simulink model "PID_controlinput_tracking"  (R2022a)
settings: Solver=VariableStepAuto  StartTime=0.0  StopTime=10  RelTol=1e-3
libraries: cstblocks x2
settings Model: Creator=Linxi Ren  LastModifiedBy=Linxi Ren

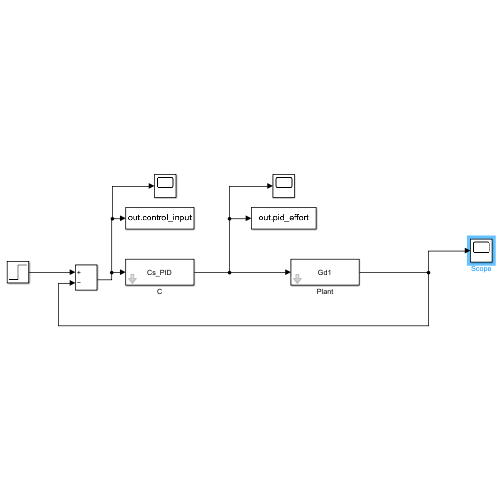
[thumbnail: Simulink's stored preview of the top-level diagram]
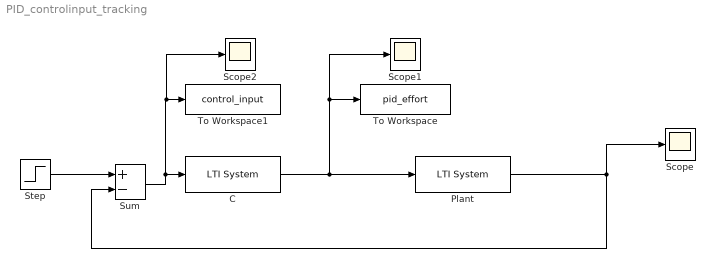
== system PID_controlinput_tracking ==
  C : cstblocks/LTI System  sys=Cs_PID  IC=[]
  Plant : cstblocks/LTI System  sys=Gd1  IC=[]
  Scope : Scope
  Scope1 : Scope
  Scope2 : Scope
  Step : Step  Time=0  SampleTime=0.0325
  Sum : Sum  Inputs=+-  InputSameDT=on  SaturateOnIntegerOverflow=on  OutDataTypeStr=Inherit: Same as first input
  To Workspace : ToWorkspace  VariableName=pid_effort  SaveFormat=Timeseries  SampleTime=-1
  To Workspace1 : ToWorkspace  VariableName=control_input  SaveFormat=Timeseries  SampleTime=-1
  wires:
  Plant/1 -> Scope/1, Sum/2
  C/1 -> Plant/1, Scope1/1, To Workspace/1
  Step/1 -> Sum/1
  Sum/1 -> Scope2/1, To Workspace1/1, C/1
